simulink model "px4Demo_FlightController_top"  (R2024a)
settings: Solver=FixedStepAuto  StartTime=0.0  StopTime=inf  RelTol=1e-3  EnableMultiTasking=on
undefined symbols (not defined in the file): SampleTime
libraries: px4uORBlib x2, px4lib x1
settings Model: ExtModeTrigDuration=10  Creator=The MathWorks, Inc.  LastModifiedBy=The MathWorks, Inc.
settings SolverCC: AlgebraicLoopSolver=TrustRegion  PositivePriorityOrder=on  MaxZcPerStep=1
settings OptimizationCC: EnhancedBackFolding=on  PassReuseOutputArgsAs=Individual arguments  ZeroExternalMemoryAtStartup=off  ZeroInternalMemoryAtStartup=off  MaxStackSize=64  OptimizeBlockOrder=speed  DifferentSizesBufferReuse=on  OptimizationCustomize=off  EfficientTunableParamExpr=on
settings DebuggingCC: ParameterTunabilityLossMsg=error  UnconnectedInputMsg=warning  UnconnectedOutputMsg=warning  UnconnectedLineMsg=warning
settings HardwareCC: ProdBitPerPointer=32  ProdBitPerSizeT=32  ProdBitPerPtrDiffT=32  ProdLargestAtomicInteger=Long  ProdLargestAtomicFloat=Double  ProdWordSize=32  ProdLongLongMode=on  ProdHWDeviceType=ARM Compatible->ARM Cortex
settings ModelReferenceCC: EnableRefExpFcnMdlSchedulingChecks=on
settings SFSimCC: MATLABDynamicMemAlloc=off  SimTargetLang=C++
settings RTWCC: Description=Embedded Coder  SystemTargetFile=ert.tlc  HardwareBoard=PX4 Host Target  TLCOptions="-aInlineSetEventsForThisBaseRateFcn=TLC_FALSE -aSuppressMultiTaskScheduler=TLC_FALSE  -aRateBasedStepFcn=0"  TemplateMakefile=ert_default_tmf  Toolchain=GNU Tools for PX4 Autopilots  PortableWordSizes=on  TargetLang=C++  GPUComputeCapability=3.5  DLArmComputeVersion=19.05
settings CodeAppCC: ForceParamTrailComments=on  IgnoreCustomStorageClasses=off  OperatorAnnotations=on  SimulinkDataObjDesc=on  SFDataObjDesc=on  InsertBlockDesc=on
settings ERTTargetCC: ExtModeTransport=2  ExtModeStaticAlloc=on  ExtModeMexFile=ext_xcp  ExtModeIntrfLevel=Level2 - Open

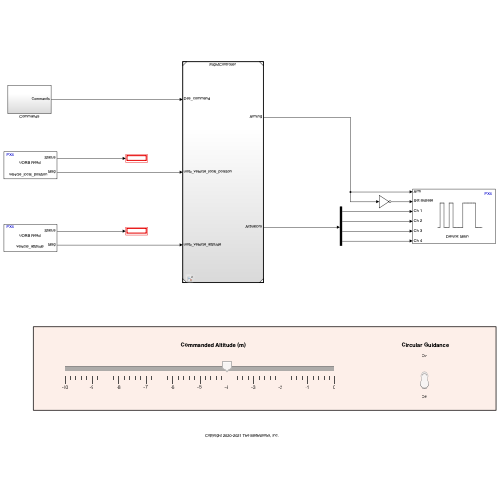
[thumbnail: Simulink's stored preview of the top-level diagram]
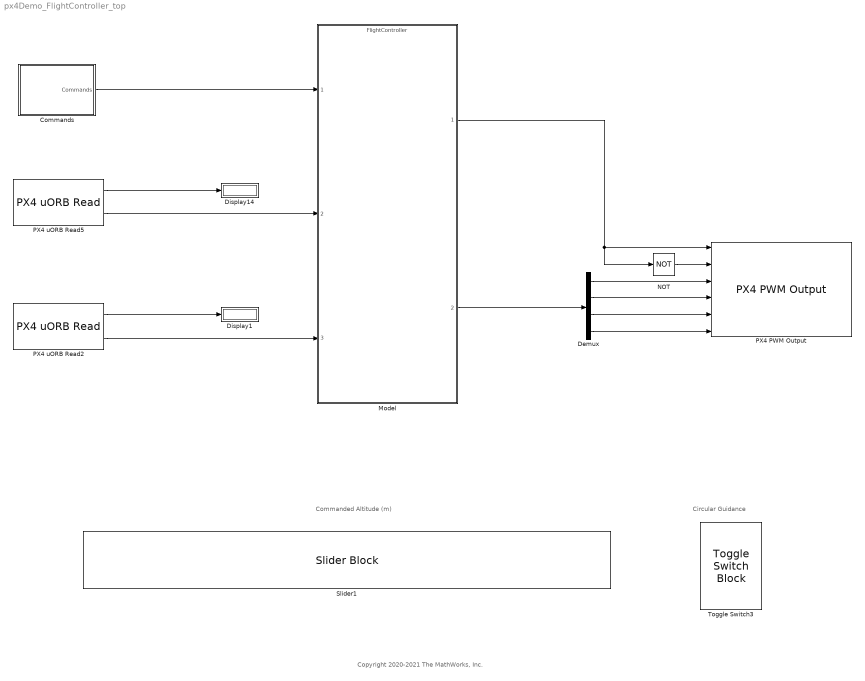
== system px4Demo_FlightController_top ==
  note: Commanded Altitude (m)
  note: Circular Guidance
  note: Copyright 2020-2021 The MathWorks, Inc.
  Commands : Subsystem
  Demux : Demux
  Display1 : Display
  Display14 : Display
  Model : ModelReference  ModelNameDialog=FlightController.slx  SimulationMode=Normal  ModelReferenceVersion=8.0
  NOT : Logic  Operator=NOT  IconShape=distinctive  AllPortsSameDT=off  OutDataTypeStr=boolean
  PX4 PWM Output : px4lib/PX4 PWM Output  pwmDevice=Main  pwmChannel1_=on  pwmChannel2_=on  pwmChannel3_=on  pwmChannel4_=on  pwmChannel5_=off  pwmChannel6_=off  pwmChannel7_=off  pwmChannel8_=off
  PX4 uORB Read2 : px4uORBlib/PX4 uORB Read  uORBTopic=vehicle_attitude  selectInstance=vehicle_attitude_groundtruth  SampleTime=SampleTime  BlockingMode=off  BlockTimeout=1e-3
  PX4 uORB Read5 : px4uORBlib/PX4 uORB Read  uORBTopic=vehicle_local_position  selectInstance=vehicle_local_position_groundtruth  SampleTime=SampleTime  BlockingMode=off  BlockTimeout=1e-3
  Slider1 : SliderBlock  LabelPosition=Hide  ScaleMin=-10  ScaleMax=0  TickInterval=1
  Toggle Switch3 : ToggleSwitchBlock  LabelPosition=Hide
      settings: Values={{'Off', 'On'}, [0 1]}
  wires:
  Commands/1(Commands) -> Model/1
  PX4 uORB Read5/1 -> Display14/1
  PX4 uORB Read2/1 -> Display1/1
  NOT/1 -> PX4 PWM Output/2
  Demux/1 -> PX4 PWM Output/3
  Demux/2 -> PX4 PWM Output/4
  Demux/3 -> PX4 PWM Output/5
  Demux/4 -> PX4 PWM Output/6
  Model/2 -> Demux/1
  Model/1 -> PX4 PWM Output/1, NOT/1
  PX4 uORB Read5/2 -> Model/2
  PX4 uORB Read2/2 -> Model/3

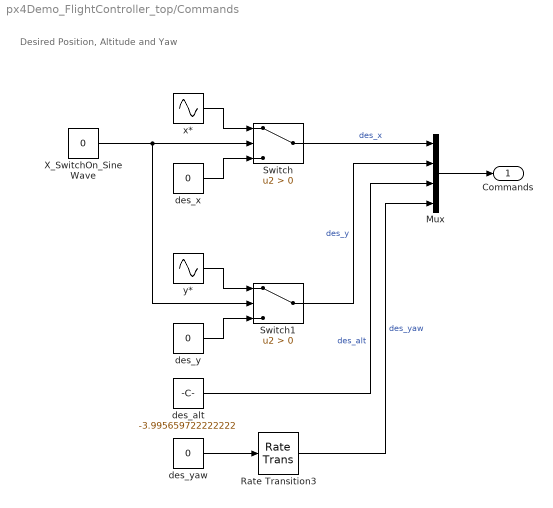
== system px4Demo_FlightController_top/Commands ==
  note: Desired Position, Altitude and Yaw
  Mux : Mux
  Rate Transition3 : RateTransition  OutPortSampleTime=SampleTime
  Switch : Switch  Criteria=u2 > Threshold  SaturateOnIntegerOverflow=off  InputSameDT=off
  Switch1 : Switch  Criteria=u2 > Threshold  SaturateOnIntegerOverflow=off  InputSameDT=off
  X_SwitchOn_Sine Wave : Constant  Value=0  SampleTime=SampleTime
  des_alt : Constant  Value=-3.995659722222222  SampleTime=SampleTime
  des_x : Constant  Value=0  SampleTime=SampleTime
  des_y : Constant  Value=0  SampleTime=SampleTime
  des_yaw : Constant  Value=0  SampleTime=SampleTime
  x* : Sin  Frequency=2*pi*.125  Phase=-pi/2  SampleTime=SampleTime
  y* : Sin  Frequency=2*pi*.125  SampleTime=SampleTime
  Commands : Outport
  wires:
  Rate Transition3/1 -> Mux/4  "des_yaw"
  des_x/1 -> Switch/3
  Switch/1 -> Mux/1  "des_x"
  Switch1/1 -> Mux/2  "des_y"
  X_SwitchOn_Sine Wave/1 -> Switch1/2, Switch/2
  des_yaw/1 -> Rate Transition3/1
  y*/1 -> Switch1/1
  des_y/1 -> Switch1/3
  x*/1 -> Switch/1
  Mux/1 -> Commands/1
  des_alt/1 -> Mux/3  "des_alt"
